simulink model "case5"  (R2024b)
settings: Solver=FixedStepAuto  StartTime=0  StopTime=1  FixedStep=1e-7  RelTol=1e-3
values from neighbouring files (symbols this model uses):
  SG_D_1_D = 0.01056    [IEEE9_case_parameters.m]    (also in case1_parameters.m; case2_parameters.m; case3_parameters.m; case4_parameters.m)
  SG_D_1_EnableSaturation = 0    [IEEE9_case_parameters.m]    (also in case1_parameters.m; case2_parameters.m; case3_parameters.m; case4_parameters.m)
  SG_D_1_f0 = 60    [IEEE9_case_parameters.m]    (also in case1_parameters.m; case2_parameters.m; case3_parameters.m; case4_parameters.m)
  SG_D_1_H = 7.5    [IEEE9_case_parameters.m]    (also in case1_parameters.m; case2_parameters.m; case3_parameters.m; case4_parameters.m)
  SG_D_1_K_A = 20    [IEEE9_case_parameters.m]    (also in case1_parameters.m; case2_parameters.m; case3_parameters.m; case4_parameters.m)
  SG_D_1_K_E = 1.000000e+1    (= 10)    [IEEE9_case_parameters.m]    (also in case1_parameters.m; case2_parameters.m; case3_parameters.m; case4_parameters.m)
  SG_D_1_K_F = 2.363    [IEEE9_case_parameters.m]    (also in case1_parameters.m; case2_parameters.m; case3_parameters.m; case4_parameters.m)
  SG_D_1_K_s = 0.5    [IEEE9_case_parameters.m]    (also in case1_parameters.m = 5; case2_parameters.m = 5; case3_parameters.m = 5; case4_parameters.m = 5)
  SG_D_1_R_a = 0.001088    [IEEE9_case_parameters.m]    (also in case1_parameters.m; case2_parameters.m; case3_parameters.m; case4_parameters.m)
  SG_D_1_S_A = 1    [IEEE9_case_parameters.m]    (also in case1_parameters.m; case2_parameters.m; case3_parameters.m; case4_parameters.m)
  SG_D_1_S_B = 0.103    [IEEE9_case_parameters.m]    (also in case1_parameters.m; case2_parameters.m; case3_parameters.m; case4_parameters.m)
  SG_D_1_S_N = 10.659857    [IEEE9_case_parameters.m]    (also in case1_parameters.m; case2_parameters.m; case3_parameters.m; case4_parameters.m)
  SG_D_1_SpeedPara = 200    [IEEE9_case_parameters.m]    (also in case1_parameters.m; case2_parameters.m; case3_parameters.m; case4_parameters.m)
  SG_D_1_T_0 = 0.720173    [IEEE9_case_parameters.m]    (also in case1_parameters.m = 0.755522; case2_parameters.m = 0.808931; case3_parameters.m = 0.869402; case4_parameters.m = 0.729316)
  SG_D_1_T_1 = 0.3    [IEEE9_case_parameters.m]    (also in case1_parameters.m; case2_parameters.m; case3_parameters.m; case4_parameters.m)
  SG_D_1_T_2 = 0.05    [IEEE9_case_parameters.m]    (also in case1_parameters.m; case2_parameters.m; case3_parameters.m; case4_parameters.m)
  SG_D_1_T_3 = 0.02    [IEEE9_case_parameters.m]    (also in case1_parameters.m; case2_parameters.m; case3_parameters.m; case4_parameters.m)
  SG_D_1_T_4 = 0.005    [IEEE9_case_parameters.m]    (also in case1_parameters.m; case2_parameters.m; case3_parameters.m; case4_parameters.m)
  SG_D_1_T_A = 0.02    [IEEE9_case_parameters.m]    (also in case1_parameters.m; case2_parameters.m; case3_parameters.m; case4_parameters.m)
  SG_D_1_T_dd = 8.000000e+0    (= 8)    [IEEE9_case_parameters.m]    (also in case1_parameters.m; case2_parameters.m; case3_parameters.m; case4_parameters.m)
  SG_D_1_T_ddd = 0.04    [IEEE9_case_parameters.m]    (also in case1_parameters.m; case2_parameters.m; case3_parameters.m; case4_parameters.m)
  SG_D_1_T_E = 0.314    [IEEE9_case_parameters.m]    (also in case1_parameters.m; case2_parameters.m; case3_parameters.m; case4_parameters.m)
  SG_D_1_T_F = 0.35    [IEEE9_case_parameters.m]    (also in case1_parameters.m; case2_parameters.m; case3_parameters.m; case4_parameters.m)
  SG_D_1_T_qd = 0.8    [IEEE9_case_parameters.m]    (also in case1_parameters.m; case2_parameters.m; case3_parameters.m; case4_parameters.m)
  SG_D_1_T_qdd = 0.02    [IEEE9_case_parameters.m]    (also in case1_parameters.m; case2_parameters.m; case3_parameters.m; case4_parameters.m)
  SG_D_1_T_speed = 0.1    [IEEE9_case_parameters.m]    (also in case1_parameters.m = 200; case2_parameters.m = 200; case3_parameters.m = 200; case4_parameters.m = 200)
  SG_D_1_T_w = 0.5    [IEEE9_case_parameters.m]    (also in case1_parameters.m; case2_parameters.m; case3_parameters.m; case4_parameters.m)
  SG_D_1_V_ref = 1.990276    [IEEE9_case_parameters.m]    (also in case1_parameters.m = 2.042296; case2_parameters.m = 2.051388; case3_parameters.m = 2.089584; case4_parameters.m = 2.01845)
  SG_D_1_w_ref = 376.991118    [IEEE9_case_parameters.m]    (also in case1_parameters.m; case2_parameters.m; case3_parameters.m; case4_parameters.m)
  SG_D_1_wb = 6.000000e+1    (= 60)    [IEEE9_case_parameters.m]    (also in case1_parameters.m; case2_parameters.m; case3_parameters.m; case4_parameters.m)
  SG_D_1_x_d = 1.9    [IEEE9_case_parameters.m]    (also in case1_parameters.m; case2_parameters.m; case3_parameters.m; case4_parameters.m)
  SG_D_1_x_dd = 0.302    [IEEE9_case_parameters.m]    (also in case1_parameters.m; case2_parameters.m; case3_parameters.m; case4_parameters.m)
  SG_D_1_x_ddd = 0.204    [IEEE9_case_parameters.m]    (also in case1_parameters.m; case2_parameters.m; case3_parameters.m; case4_parameters.m)
  SG_D_1_x_l = 0.05    [IEEE9_case_parameters.m]    (also in case1_parameters.m; case2_parameters.m; case3_parameters.m; case4_parameters.m)
  SG_D_1_x_q = 1.3    [IEEE9_case_parameters.m]    (also in case1_parameters.m; case2_parameters.m; case3_parameters.m; case4_parameters.m)
  SG_D_1_x_qd = 0.5    [IEEE9_case_parameters.m]    (also in case1_parameters.m; case2_parameters.m; case3_parameters.m; case4_parameters.m)
  SG_D_1_x_qdd = 0.3    [IEEE9_case_parameters.m]    (also in case1_parameters.m; case2_parameters.m; case3_parameters.m; case4_parameters.m)
  SG_D_2_D = 0.02    [IEEE9_case_parameters.m]    (also in case1_parameters.m; case2_parameters.m; case3_parameters.m; case4_parameters.m)
  SG_D_2_EnableSaturation = 0    [IEEE9_case_parameters.m]    (also in case1_parameters.m; case2_parameters.m; case3_parameters.m; case4_parameters.m)
  SG_D_2_f0 = 60    [IEEE9_case_parameters.m]    (also in case1_parameters.m; case2_parameters.m; case3_parameters.m; case4_parameters.m)
  SG_D_2_H = 8.000000e+0    (= 8)    [IEEE9_case_parameters.m]    (also in case1_parameters.m; case2_parameters.m; case3_parameters.m; case4_parameters.m)
  SG_D_2_K_A = 20    [IEEE9_case_parameters.m]    (also in case1_parameters.m; case2_parameters.m; case3_parameters.m; case4_parameters.m)
  SG_D_2_K_E = 1.000000e+1    (= 10)    [IEEE9_case_parameters.m]    (also in case1_parameters.m; case2_parameters.m; case3_parameters.m; case4_parameters.m)
  SG_D_2_K_F = 2.363    [IEEE9_case_parameters.m]    (also in case1_parameters.m; case2_parameters.m; case3_parameters.m; case4_parameters.m)
  SG_D_2_K_s = 0.5    [IEEE9_case_parameters.m]    (also in case1_parameters.m = 4; case2_parameters.m = 4; case3_parameters.m = 4; case4_parameters.m = 4)
  SG_D_2_R_a = 0.001088    [IEEE9_case_parameters.m]    (also in case1_parameters.m; case2_parameters.m; case3_parameters.m; case4_parameters.m)
  SG_D_2_S_A = 1    [IEEE9_case_parameters.m]    (also in case1_parameters.m; case2_parameters.m; case3_parameters.m; case4_parameters.m)
  SG_D_2_S_B = 0.103    [IEEE9_case_parameters.m]    (also in case1_parameters.m; case2_parameters.m; case3_parameters.m; case4_parameters.m)
  SG_D_2_S_N = 10.659857    [IEEE9_case_parameters.m]    (also in case1_parameters.m; case2_parameters.m; case3_parameters.m; case4_parameters.m)
  SG_D_2_SpeedPara = 200    [IEEE9_case_parameters.m]    (also in case1_parameters.m; case2_parameters.m; case3_parameters.m; case4_parameters.m)
  SG_D_2_T_0 = 1.632913    [IEEE9_case_parameters.m]    (also in case1_parameters.m = 1.632925; case2_parameters.m = 1.632915; case3_parameters.m = 1.632914; case4_parameters.m = 1.632927)
  SG_D_2_T_1 = 0.2    [IEEE9_case_parameters.m]    (also in case1_parameters.m; case2_parameters.m; case3_parameters.m; case4_parameters.m)
  SG_D_2_T_2 = 0.05    [IEEE9_case_parameters.m]    (also in case1_parameters.m; case2_parameters.m; case3_parameters.m; case4_parameters.m)
  SG_D_2_T_3 = 0.02    [IEEE9_case_parameters.m]    (also in case1_parameters.m; case2_parameters.m; case3_parameters.m; case4_parameters.m)
  SG_D_2_T_4 = 0.005    [IEEE9_case_parameters.m]    (also in case1_parameters.m; case2_parameters.m; case3_parameters.m; case4_parameters.m)
  SG_D_2_T_A = 0.02    [IEEE9_case_parameters.m]    (also in case1_parameters.m; case2_parameters.m; case3_parameters.m; case4_parameters.m)
  SG_D_2_T_dd = 7.9    [IEEE9_case_parameters.m]    (also in case1_parameters.m; case2_parameters.m; case3_parameters.m; case4_parameters.m)
  SG_D_2_T_ddd = 0.04    [IEEE9_case_parameters.m]    (also in case1_parameters.m; case2_parameters.m; case3_parameters.m; case4_parameters.m)
  SG_D_2_T_E = 0.314    [IEEE9_case_parameters.m]    (also in case1_parameters.m; case2_parameters.m; case3_parameters.m; case4_parameters.m)
  SG_D_2_T_F = 0.35    [IEEE9_case_parameters.m]    (also in case1_parameters.m; case2_parameters.m; case3_parameters.m; case4_parameters.m)
  SG_D_2_T_qd = 0.8    [IEEE9_case_parameters.m]    (also in case1_parameters.m; case2_parameters.m; case3_parameters.m; case4_parameters.m)
  SG_D_2_T_qdd = 0.015    [IEEE9_case_parameters.m]    (also in case1_parameters.m; case2_parameters.m; case3_parameters.m; case4_parameters.m)
  SG_D_2_T_speed = 0.1    [IEEE9_case_parameters.m]    (also in case1_parameters.m = 150; case2_parameters.m = 150; case3_parameters.m = 150; case4_parameters.m = 150)
  SG_D_2_T_w = 0.35    [IEEE9_case_parameters.m]    (also in case1_parameters.m; case2_parameters.m; case3_parameters.m; case4_parameters.m)
  SG_D_2_V_ref = 2.58547    [IEEE9_case_parameters.m]    (also in case1_parameters.m = 2.597896; case2_parameters.m = 2.587136; case3_parameters.m = 2.586042; case4_parameters.m = 2.599679)
  SG_D_2_w_ref = 376.991118    [IEEE9_case_parameters.m]    (also in case1_parameters.m; case2_parameters.m; case3_parameters.m; case4_parameters.m)
  SG_D_2_wb = 6.000000e+1    (= 60)    [IEEE9_case_parameters.m]    (also in case1_parameters.m; case2_parameters.m; case3_parameters.m; case4_parameters.m)
  SG_D_2_x_d = 1.8    [IEEE9_case_parameters.m]    (also in case1_parameters.m; case2_parameters.m; case3_parameters.m; case4_parameters.m)
  SG_D_2_x_dd = 0.302    [IEEE9_case_parameters.m]    (also in case1_parameters.m; case2_parameters.m; case3_parameters.m; case4_parameters.m)
  SG_D_2_x_ddd = 0.204    [IEEE9_case_parameters.m]    (also in case1_parameters.m; case2_parameters.m; case3_parameters.m; case4_parameters.m)
  SG_D_2_x_l = 0.05    [IEEE9_case_parameters.m]    (also in case1_parameters.m; case2_parameters.m; case3_parameters.m; case4_parameters.m)
  SG_D_2_x_q = 1.25    [IEEE9_case_parameters.m]    (also in case1_parameters.m; case2_parameters.m; case3_parameters.m; case4_parameters.m)
  SG_D_2_x_qd = 0.5    [IEEE9_case_parameters.m]    (also in case1_parameters.m; case2_parameters.m; case3_parameters.m; case4_parameters.m)
  SG_D_2_x_qdd = 0.3    [IEEE9_case_parameters.m]    (also in case1_parameters.m; case2_parameters.m; case3_parameters.m; case4_parameters.m)
  SG_D_3_D = 0.02    [IEEE9_case_parameters.m]    (also in case1_parameters.m; case2_parameters.m; case3_parameters.m; case4_parameters.m)
  SG_D_3_EnableSaturation = 0    [IEEE9_case_parameters.m]    (also in case1_parameters.m; case2_parameters.m; case3_parameters.m; case4_parameters.m)
  SG_D_3_f0 = 60    [IEEE9_case_parameters.m]    (also in case1_parameters.m; case2_parameters.m; case3_parameters.m; case4_parameters.m)
  SG_D_3_H = 7.7    [IEEE9_case_parameters.m]    (also in case1_parameters.m; case2_parameters.m; case3_parameters.m; case4_parameters.m)
  SG_D_3_K_A = 20    [IEEE9_case_parameters.m]    (also in case1_parameters.m; case2_parameters.m; case3_parameters.m; case4_parameters.m)
  SG_D_3_K_E = 1.000000e+1    (= 10)    [IEEE9_case_parameters.m]    (also in case1_parameters.m; case2_parameters.m; case3_parameters.m; case4_parameters.m)
  SG_D_3_K_F = 2.363    [IEEE9_case_parameters.m]    (also in case1_parameters.m; case2_parameters.m; case3_parameters.m; case4_parameters.m)
  SG_D_3_K_s = 0.2    [IEEE9_case_parameters.m]    (also in case1_parameters.m = 2; case2_parameters.m = 2; case3_parameters.m = 2; case4_parameters.m = 2)
  SG_D_3_R_a = 0.001088    [IEEE9_case_parameters.m]    (also in case1_parameters.m; case2_parameters.m; case3_parameters.m; case4_parameters.m)
  SG_D_3_S_A = 1    [IEEE9_case_parameters.m]    (also in case1_parameters.m; case2_parameters.m; case3_parameters.m; case4_parameters.m)
  SG_D_3_S_B = 0.103    [IEEE9_case_parameters.m]    (also in case1_parameters.m; case2_parameters.m; case3_parameters.m; case4_parameters.m)
  SG_D_3_S_N = 10.659857    [IEEE9_case_parameters.m]    (also in case1_parameters.m; case2_parameters.m; case3_parameters.m; case4_parameters.m)
  SG_D_3_SpeedPara = 200    [IEEE9_case_parameters.m]    (also in case1_parameters.m; case2_parameters.m; case3_parameters.m; case4_parameters.m)
  SG_D_3_T_0 = 0.850788    [IEEE9_case_parameters.m]    (also in case1_parameters.m = 0.850786; case2_parameters.m = 0.850787; case3_parameters.m; case4_parameters.m = 0.850786)
  SG_D_3_T_1 = 0.2    [IEEE9_case_parameters.m]    (also in case1_parameters.m; case2_parameters.m; case3_parameters.m; case4_parameters.m)
  SG_D_3_T_2 = 0.05    [IEEE9_case_parameters.m]    (also in case1_parameters.m; case2_parameters.m; case3_parameters.m; case4_parameters.m)
  SG_D_3_T_3 = 0.02    [IEEE9_case_parameters.m]    (also in case1_parameters.m; case2_parameters.m; case3_parameters.m; case4_parameters.m)
  SG_D_3_T_4 = 0.005    [IEEE9_case_parameters.m]    (also in case1_parameters.m; case2_parameters.m; case3_parameters.m; case4_parameters.m)
  SG_D_3_T_A = 0.02    [IEEE9_case_parameters.m]    (also in case1_parameters.m; case2_parameters.m; case3_parameters.m; case4_parameters.m)
  SG_D_3_T_dd = 8.1    [IEEE9_case_parameters.m]    (also in case1_parameters.m; case2_parameters.m; case3_parameters.m; case4_parameters.m)
  SG_D_3_T_ddd = 0.04    [IEEE9_case_parameters.m]    (also in case1_parameters.m; case2_parameters.m; case3_parameters.m; case4_parameters.m)
  SG_D_3_T_E = 0.314    [IEEE9_case_parameters.m]    (also in case1_parameters.m; case2_parameters.m; case3_parameters.m; case4_parameters.m)
  SG_D_3_T_F = 0.35    [IEEE9_case_parameters.m]    (also in case1_parameters.m; case2_parameters.m; case3_parameters.m; case4_parameters.m)
  SG_D_3_T_qd = 0.8    [IEEE9_case_parameters.m]    (also in case1_parameters.m; case2_parameters.m; case3_parameters.m; case4_parameters.m)
  SG_D_3_T_qdd = 0.015    [IEEE9_case_parameters.m]    (also in case1_parameters.m; case2_parameters.m; case3_parameters.m; case4_parameters.m)
  SG_D_3_T_speed = 0.1    [IEEE9_case_parameters.m]    (also in case1_parameters.m = 180; case2_parameters.m = 180; case3_parameters.m = 180; case4_parameters.m = 180)
  SG_D_3_T_w = 0.4    [IEEE9_case_parameters.m]    (also in case1_parameters.m; case2_parameters.m; case3_parameters.m; case4_parameters.m)
  SG_D_3_V_ref = 1.892727    [IEEE9_case_parameters.m]    (also in case1_parameters.m = 1.906439; case2_parameters.m = 1.895535; case3_parameters.m = 1.892105; case4_parameters.m = 1.906598)
  SG_D_3_w_ref = 376.991118    [IEEE9_case_parameters.m]    (also in case1_parameters.m; case2_parameters.m; case3_parameters.m; case4_parameters.m)
  SG_D_3_wb = 6.000000e+1    (= 60)    [IEEE9_case_parameters.m]    (also in case1_parameters.m; case2_parameters.m; case3_parameters.m; case4_parameters.m)
  SG_D_3_x_d = 1.85    [IEEE9_case_parameters.m]    (also in case1_parameters.m; case2_parameters.m; case3_parameters.m; case4_parameters.m)
  SG_D_3_x_dd = 0.302    [IEEE9_case_parameters.m]    (also in case1_parameters.m; case2_parameters.m; case3_parameters.m; case4_parameters.m)
  SG_D_3_x_ddd = 0.204    [IEEE9_case_parameters.m]    (also in case1_parameters.m; case2_parameters.m; case3_parameters.m; case4_parameters.m)
  SG_D_3_x_l = 0.05    [IEEE9_case_parameters.m]    (also in case1_parameters.m; case2_parameters.m; case3_parameters.m; case4_parameters.m)
  SG_D_3_x_q = 1.2    [IEEE9_case_parameters.m]    (also in case1_parameters.m; case2_parameters.m; case3_parameters.m; case4_parameters.m)
  SG_D_3_x_qd = 0.5    [IEEE9_case_parameters.m]    (also in case1_parameters.m; case2_parameters.m; case3_parameters.m; case4_parameters.m)
  SG_D_3_x_qdd = 0.3    [IEEE9_case_parameters.m]    (also in case1_parameters.m; case2_parameters.m; case3_parameters.m; case4_parameters.m)
(part 8 of 12)

== system case5/SG_D_2/d_psi_d_SG_D_2_block ==
  note: d_psi_d_SG_D_2 in case5
      | $2\,\pi \,f_{0}\,\left(v_{d,\mathrm{SG},D,2}\,\sin\left(\theta _{\mathrm{SG},D,2}\right)-v_{q,\mathrm{SG},D,2}\,\cos\left(\theta _{\mathrm{SG},D,2}\right)+\frac{R_{a}\,\left(\frac{\psi _{\mathrm{1d},\mathrm{SG},D,2}\,\left(x_{\mathrm{dd}}-x_{\mathrm{ddd}}\right)}{x_{\mathrm{dd}}-x_{l}}-\psi _{d,\mathrm{SG},D,2}+\frac{\psi _{\mathrm{fd},\mathrm{SG},D,2}\,\left(x_{\mathrm{ddd}}-x_{l}\right)}{x_{\mathrm{dd}}-x_{l}}\right)}{x_{\mathrm{ddd}}}+\frac{\psi _{q,\mathrm{SG},D,2}\,w_{\mathrm{SG},D,2}}{2\,f_{0}\,\pi }\right)$
      | Automatically generated on 2025-10-31 19:10:55 .
  State_psi_1d_SG_D_2_04eff : Inport
  State_psi_d_SG_D_2_38234 : Inport  Port=2
  State_psi_fd_SG_D_2_ff9ed : Inport  Port=3
  Input_v_d_SG_D_2_e8182 : Inport  Port=4
  State_theta_SG_D_2_47dce : Inport  Port=5
  Input_v_q_SG_D_2_617bb : Inport  Port=6
  State_theta_SG_D_2_18c28 : Inport  Port=7
  State_psi_q_SG_D_2_39081 : Inport  Port=8
  State_w_SG_D_2_93911 : Inport  Port=9
  Add_35a87 : Sum
  Add_8a6e8 : Sum
  Constant_-1_40228 : Constant  Value=-1
  Constant_-2.0_2b37e : Constant  Value=-2.0
  Constant_2.0_61fa9 : Constant  Value=2.0
  Constant_R_a_dc03f : Constant  Value=R_a
  Constant_f0_9e30f : Constant  Value=f0
  Constant_f0_ea738 : Constant  Value=f0
  Constant_pi_80db8 : Constant  Value=pi
  Constant_pi_cc7e5 : Constant  Value=pi
  Constant_x_dd_383e0 : Constant  Value=x_dd
  Constant_x_dd_5a803 : Constant  Value=x_dd
  Constant_x_dd_d00b2 : Constant  Value=x_dd
  Constant_x_ddd_020f5 : Constant  Value=x_ddd
  Constant_x_ddd_24d94 : Constant  Value=x_ddd
  Constant_x_ddd_dd370 : Constant  Value=x_ddd
  Constant_x_l_7a989 : Constant  Value=x_l
  Constant_x_l_d2dea : Constant  Value=x_l
  Constant_x_l_e9755 : Constant  Value=x_l
  Divide_2b41b : Product  Inputs=*/
  Divide_53e77 : Product  Inputs=*/
  Divide_973af : Product  Inputs=*/
  Divide_a5896 : Product  Inputs=*/
  MathFunc_cos_96fd6 : Trigonometry  Operator=cos
  MathFunc_sin_6bfeb : Trigonometry
  Product_21970 : Product
  Product_5265e : Product
  Product_60fe7 : Product
  Product_61b83 : Product
  Product_79863 : Product
  Product_8e8bd : Product
  Product_ab31f : Product
  Product_caa64 : Product
  Product_cea4f : Product
  Product_d6891 : Product
  Product_e49bf : Product
  Product_fc14d : Product
  Subtract_54247 : Sum  Inputs=+-
  Subtract_54db2 : Sum  Inputs=+-
  Subtract_7347e : Sum  Inputs=+-
  Subtract_9dfb5 : Sum  Inputs=+-
  Subtract_e25de : Sum  Inputs=+-
  Subtract_e48e5 : Sum  Inputs=+-
  Subtract_f9a11 : Sum  Inputs=+-
  Blockout_d_psi_d_SG_D_2_c5ec0 : Outport
  wires:
  MathFunc_sin_6bfeb/1 -> Product_d6891/2
  Constant_x_dd_d00b2/1 -> Subtract_9dfb5/1
  Constant_-1_40228/1 -> Product_8e8bd/1
  Constant_x_l_d2dea/1 -> Subtract_9dfb5/2
  State_psi_1d_SG_D_2_04eff/1 -> Product_8e8bd/2
  Constant_f0_ea738/1 -> Product_5265e/2
  Constant_2.0_61fa9/1 -> Product_e49bf/1
  Constant_x_l_e9755/1 -> Subtract_f9a11/2
  Constant_x_dd_5a803/1 -> Subtract_54db2/1
  Product_60fe7/1 -> Blockout_d_psi_d_SG_D_2_c5ec0/1
  Constant_pi_cc7e5/1 -> Product_e49bf/2
  Constant_x_ddd_020f5/1 -> Subtract_54db2/2
  Subtract_e48e5/1 -> Product_60fe7/2
  Product_8e8bd/1 -> Product_caa64/1
  Product_e49bf/1 -> Product_61b83/1
  Subtract_54db2/1 -> Product_caa64/2
  Divide_a5896/1 -> Subtract_e48e5/2
  Constant_x_ddd_24d94/1 -> Subtract_e25de/1
  Constant_x_l_7a989/1 -> Subtract_e25de/2
  Product_caa64/1 -> Divide_53e77/1
  Subtract_54247/1 -> Add_8a6e8/1
  Subtract_9dfb5/1 -> Divide_53e77/2
  State_psi_fd_SG_D_2_ff9ed/1 -> Product_fc14d/1
  Subtract_e25de/1 -> Product_fc14d/2
  Constant_x_dd_383e0/1 -> Subtract_f9a11/1
  Divide_53e77/1 -> Add_35a87/1
  State_psi_d_SG_D_2_38234/1 -> Add_35a87/2
  Product_fc14d/1 -> Divide_2b41b/1
  Subtract_f9a11/1 -> Divide_2b41b/2
  Add_35a87/1 -> Subtract_7347e/1
  Divide_2b41b/1 -> Subtract_7347e/2
  Constant_R_a_dc03f/1 -> Product_ab31f/1
  Subtract_7347e/1 -> Product_ab31f/2
  Divide_973af/1 -> Subtract_54247/1
  State_theta_SG_D_2_47dce/1 -> MathFunc_sin_6bfeb/1
  Product_ab31f/1 -> Divide_973af/1
  Constant_-2.0_2b37e/1 -> Product_79863/1
  Input_v_d_SG_D_2_e8182/1 -> Product_d6891/1
  Constant_x_ddd_dd370/1 -> Divide_973af/2
  State_theta_SG_D_2_18c28/1 -> MathFunc_cos_96fd6/1
  Product_5265e/1 -> Product_60fe7/1
  Product_d6891/1 -> Subtract_54247/2
  Product_79863/1 -> Product_5265e/1
  Input_v_q_SG_D_2_617bb/1 -> Product_cea4f/1
  MathFunc_cos_96fd6/1 -> Product_cea4f/2
  State_psi_q_SG_D_2_39081/1 -> Product_21970/1
  State_w_SG_D_2_93911/1 -> Product_21970/2
  Constant_f0_9e30f/1 -> Product_61b83/2
  Constant_pi_80db8/1 -> Product_79863/2
  Product_cea4f/1 -> Add_8a6e8/2
  Product_21970/1 -> Divide_a5896/1
  Product_61b83/1 -> Divide_a5896/2
  Add_8a6e8/1 -> Subtract_e48e5/1

== system case5/SG_D_2/d_psi_fd_SG_D_2_block ==
  note: d_psi_fd_SG_D_2 in case5
      | $-\frac{\psi _{\mathrm{fd},\mathrm{SG},D,2}-E_{\mathrm{fd},\mathrm{SG},D,2}+\left(x_{d}-x_{\mathrm{dd}}\right)\,\left(\frac{\frac{\psi _{\mathrm{1d},\mathrm{SG},D,2}\,\left(x_{\mathrm{dd}}-x_{\mathrm{ddd}}\right)}{x_{\mathrm{dd}}-x_{l}}-\psi _{d,\mathrm{SG},D,2}+\frac{\psi _{\mathrm{fd},\mathrm{SG},D,2}\,\left(x_{\mathrm{ddd}}-x_{l}\right)}{x_{\mathrm{dd}}-x_{l}}}{x_{\mathrm{ddd}}}-\frac{\left(x_{\mathrm{dd}}-x_{\mathrm{ddd}}\right)\,\left(\psi _{\mathrm{1d},\mathrm{SG},D,2}-\psi _{\mathrm{fd},\mathrm{SG},D,2}+\frac{\left(x_{\mathrm{dd}}-x_{l}\right)\,\left(\frac{\psi _{\mathrm{1d},\mathrm{SG},D,2}\,\left(x_{\mathrm{dd}}-x_{\mathrm{ddd}}\right)}{x_{\mathrm{dd}}-x_{l}}-\psi _{d,\mathrm{SG},D,2}+\frac{\psi _{\mathrm{fd},\mathrm{SG},D,2}\,\left(x_{\mathrm{ddd}}-x_{l}\right)}{x_{\mathrm{dd}}-x_{l}}\right)}{x_{\mathrm{ddd}}}\right)}{{\left(x_{\mathrm{dd}}-x_{l}\right)}^2}\right)}{T_{\mathrm{dd}}}$
      | Automatically generated on 2025-10-31 19:11:05 .
  State_E_fd_SG_D_2_4bfea : Inport
  State_psi_fd_SG_D_2_52249 : Inport  Port=2
  State_psi_1d_SG_D_2_569a8 : Inport  Port=3
  State_psi_fd_SG_D_2_bd521 : Inport  Port=4
  State_psi_1d_SG_D_2_de869 : Inport  Port=5
  State_psi_d_SG_D_2_2ae43 : Inport  Port=6
  State_psi_fd_SG_D_2_2448d : Inport  Port=7
  State_psi_1d_SG_D_2_50b72 : Inport  Port=8
  State_psi_d_SG_D_2_60bb1 : Inport  Port=9
  State_psi_fd_SG_D_2_29cbb : Inport  Port=10
  Add_807b0 : Sum
  Add_92990 : Sum
  Constant_-1_18d3b : Constant  Value=-1
  Constant_-1_23845 : Constant  Value=-1
  Constant_-1_3a1c2 : Constant  Value=-1
  Constant_2.0_fae6e : Constant  Value=2.0
  Constant_T_dd_c2c29 : Constant  Value=T_dd
  Constant_x_d_43747 : Constant  Value=x_d
  Constant_x_dd_10bf3 : Constant  Value=x_dd
  Constant_x_dd_24d9e : Constant  Value=x_dd
  Constant_x_dd_261bc : Constant  Value=x_dd
  Constant_x_dd_4acb3 : Constant  Value=x_dd
  Constant_x_dd_c1aff : Constant  Value=x_dd
  Constant_x_dd_cff65 : Constant  Value=x_dd
  Constant_x_dd_d5cdf : Constant  Value=x_dd
  Constant_x_dd_dae7c : Constant  Value=x_dd
  Constant_x_dd_f7268 : Constant  Value=x_dd
  Constant_x_dd_fe35d : Constant  Value=x_dd
  Constant_x_ddd_0888f : Constant  Value=x_ddd
  Constant_x_ddd_124ec : Constant  Value=x_ddd
  Constant_x_ddd_44805 : Constant  Value=x_ddd
  Constant_x_ddd_7c7c3 : Constant  Value=x_ddd
  Constant_x_ddd_a1edb : Constant  Value=x_ddd
  Constant_x_ddd_a6cd1 : Constant  Value=x_ddd
  Constant_x_ddd_c2edf : Constant  Value=x_ddd
  Constant_x_l_59093 : Constant  Value=x_l
  Constant_x_l_768d7 : Constant  Value=x_l
  Constant_x_l_7bddd : Constant  Value=x_l
  Constant_x_l_92fb9 : Constant  Value=x_l
  Constant_x_l_b5f95 : Constant  Value=x_l
  Constant_x_l_ca421 : Constant  Value=x_l
  Constant_x_l_cff4a : Constant  Value=x_l
  Constant_x_l_d3abc : Constant  Value=x_l
  Divide_46224 : Product  Inputs=*/
  Divide_4a4ac : Product  Inputs=*/
  Divide_67d0a : Product  Inputs=*/
  Divide_6e8e2 : Product  Inputs=*/
  Divide_7626a : Product  Inputs=*/
  Divide_8d5c8 : Product  Inputs=*/
  Divide_c3267 : Product  Inputs=*/
  Divide_c3f1b : Product  Inputs=*/
  Power_391a0 : Math  Operator=pow
  Product_271b3 : Product
  Product_461f0 : Product
  Product_624bd : Product
  Product_95ff3 : Product
  Product_b9362 : Product
  Product_baa0b : Product
  Product_d2126 : Product
  Product_eaf31 : Product
  Product_f9a51 : Product
  Product_ff220 : Product
  Subtract_01693 : Sum  Inputs=+-
  Subtract_099c9 : Sum  Inputs=+-
  Subtract_0f381 : Sum  Inputs=+-
  Subtract_17e32 : Sum  Inputs=+-
  Subtract_25243 : Sum  Inputs=+-
  Subtract_283d9 : Sum  Inputs=+-
  Subtract_2ee32 : Sum  Inputs=+-
  Subtract_301a9 : Sum  Inputs=+-
  Subtract_3e025 : Sum  Inputs=+-
  Subtract_74e66 : Sum  Inputs=+-
  Subtract_79f9a : Sum  Inputs=+-
  Subtract_8fe35 : Sum  Inputs=+-
  Subtract_9ac67 : Sum  Inputs=+-
  Subtract_ab91b : Sum  Inputs=+-
  Subtract_b343b : Sum  Inputs=+-
  Subtract_bbb0c : Sum  Inputs=+-
  Subtract_d8d56 : Sum  Inputs=+-
  Subtract_dd31b : Sum  Inputs=+-
  Subtract_e919c : Sum  Inputs=+-
  Blockout_d_psi_fd_SG_D_2_6ca49 : Outport
  wires:
  Constant_x_dd_cff65/1 -> Subtract_b343b/1
  Constant_-1_3a1c2/1 -> Product_eaf31/1
  Constant_x_l_d3abc/1 -> Subtract_ab91b/2
  Divide_46224/1 -> Add_807b0/1
  Subtract_099c9/1 -> Product_ff220/2
  Constant_x_l_768d7/1 -> Subtract_b343b/2
  Product_ff220/1 -> Divide_4a4ac/1
  State_psi_1d_SG_D_2_de869/1 -> Product_eaf31/2
  Constant_x_dd_f7268/1 -> Subtract_2ee32/1
  Product_461f0/1 -> Divide_46224/1
  Constant_x_dd_d5cdf/1 -> Subtract_0f381/1
  Constant_x_ddd_124ec/1 -> Subtract_2ee32/2
  Constant_x_dd_261bc/1 -> Subtract_dd31b/1
  Product_eaf31/1 -> Product_b9362/1
  Subtract_2ee32/1 -> Product_b9362/2
  State_psi_d_SG_D_2_60bb1/1 -> Add_807b0/2
  Constant_x_ddd_a1edb/1 -> Subtract_099c9/1
  Constant_x_l_59093/1 -> Subtract_099c9/2
  Product_b9362/1 -> Divide_c3267/1
  Subtract_b343b/1 -> Divide_c3267/2
  State_psi_fd_SG_D_2_2448d/1 -> Product_ff220/1
  Subtract_79f9a/1 -> Product_d2126/2
  Constant_x_dd_24d9e/1 -> Subtract_e919c/1
  Constant_x_l_7bddd/1 -> Subtract_e919c/2
  Product_624bd/1 -> Product_d2126/1
  Divide_c3267/1 -> Add_92990/1
  State_psi_d_SG_D_2_2ae43/1 -> Add_92990/2
  Subtract_e919c/1 -> Divide_4a4ac/2
  Constant_x_dd_fe35d/1 -> Subtract_ab91b/1
  Constant_x_ddd_a6cd1/1 -> Subtract_01693/1
  Add_92990/1 -> Subtract_17e32/1
  Divide_4a4ac/1 -> Subtract_17e32/2
  Constant_-1_23845/1 -> Product_baa0b/1
  Product_95ff3/1 -> Divide_7626a/1
  State_psi_1d_SG_D_2_50b72/1 -> Product_baa0b/2
  Subtract_0f381/1 -> Product_624bd/2
  Constant_x_dd_4acb3/1 -> Subtract_d8d56/1
  Divide_7626a/1 -> Subtract_8fe35/2
  Constant_-1_18d3b/1 -> Product_624bd/1
  Constant_x_ddd_c2edf/1 -> Subtract_d8d56/2
  Constant_x_ddd_0888f/1 -> Divide_6e8e2/2
  Subtract_ab91b/1 -> Product_271b3/1
  Subtract_17e32/1 -> Product_271b3/2
  State_psi_fd_SG_D_2_bd521/1 -> Subtract_9ac67/2
  Product_baa0b/1 -> Product_461f0/1
  Subtract_d8d56/1 -> Product_461f0/2
  Constant_2.0_fae6e/1 -> Power_391a0/2
  State_psi_1d_SG_D_2_569a8/1 -> Subtract_9ac67/1
  Constant_x_dd_dae7c/1 -> Subtract_301a9/1
  Subtract_01693/1 -> Product_95ff3/2
  Constant_x_l_ca421/1 -> Subtract_301a9/2
  Constant_x_l_cff4a/1 -> Subtract_01693/2
  Constant_x_ddd_44805/1 -> Subtract_0f381/2
  Subtract_dd31b/1 -> Divide_7626a/2
  Product_271b3/1 -> Divide_6e8e2/1
  Subtract_301a9/1 -> Divide_46224/2
  State_psi_fd_SG_D_2_29cbb/1 -> Product_95ff3/1
  Constant_x_l_b5f95/1 -> Subtract_dd31b/2
  Constant_x_dd_10bf3/1 -> Subtract_bbb0c/1
  Subtract_9ac67/1 -> Subtract_79f9a/1
  Divide_6e8e2/1 -> Subtract_79f9a/2
  Constant_x_l_92fb9/1 -> Subtract_bbb0c/2
  Subtract_bbb0c/1 -> Power_391a0/1
  Add_807b0/1 -> Subtract_8fe35/1
  Product_d2126/1 -> Divide_c3f1b/1
  Power_391a0/1 -> Divide_c3f1b/2
  Subtract_8fe35/1 -> Divide_8d5c8/1
  Constant_x_ddd_7c7c3/1 -> Divide_8d5c8/2
  Constant_x_d_43747/1 -> Subtract_25243/1
  Constant_x_dd_c1aff/1 -> Subtract_25243/2
  Divide_c3f1b/1 -> Subtract_283d9/1
  Divide_8d5c8/1 -> Subtract_283d9/2
  State_E_fd_SG_D_2_4bfea/1 -> Subtract_3e025/1
  State_psi_fd_SG_D_2_52249/1 -> Subtract_3e025/2
  Subtract_25243/1 -> Product_f9a51/1
  Subtract_283d9/1 -> Product_f9a51/2
  Subtract_3e025/1 -> Subtract_74e66/1
  Product_f9a51/1 -> Subtract_74e66/2
  Subtract_74e66/1 -> Divide_67d0a/1
  Constant_T_dd_c2c29/1 -> Divide_67d0a/2
  Divide_67d0a/1 -> Blockout_d_psi_fd_SG_D_2_6ca49/1

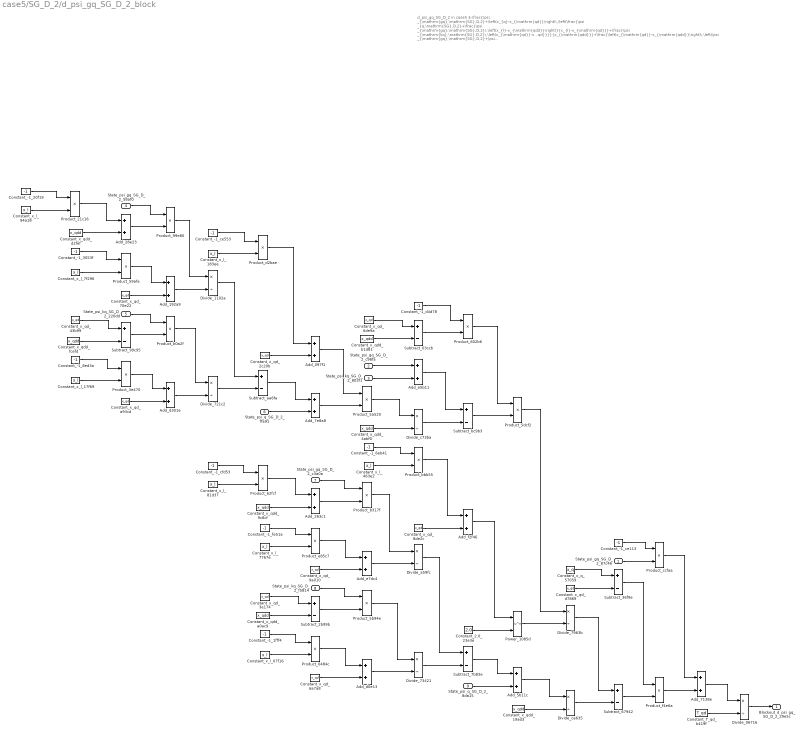
== system case5/SG_D_2/d_psi_gq_SG_D_2_block ==
  note: d_psi_gq_SG_D_2 in case5
      | $-\frac{\psi _{\mathrm{gq},\mathrm{SG},D,2}+\left(x_{q}-x_{\mathrm{qd}}\right)\,\left(\frac{\psi _{q,\mathrm{SG},D,2}+\frac{\psi _{\mathrm{gq},\mathrm{SG},D,2}\,\left(x_{l}-x_{\mathrm{qdd}}\right)}{x_{l}-x_{\mathrm{qd}}}+\frac{\psi _{\mathrm{kq},\mathrm{SG},D,2}\,\left(x_{\mathrm{qd}}-x_{\mathrm{qdd}}\right)}{x_{l}-x_{\mathrm{qd}}}}{x_{\mathrm{qdd}}}+\frac{\left(x_{\mathrm{qd}}-x_{\mathrm{qdd}}\right)\,\left(\psi _{\mathrm{gq},\mathrm{SG},D,2}+\psi _{\mathrm{kq},\mathrm{SG},D,2}+\frac{\left(x_{l}-x_{\mathrm{qd}}\right)\,\left(\psi _{q,\mathrm{SG},D,2}+\frac{\psi _{\mathrm{gq},\mathrm{SG},D,2}\,\left(x_{l}-x_{\mathrm{qdd}}\right)}{x_{l}-x_{\mathrm{qd}}}+\frac{\psi _{\mathrm{kq},\mathrm{SG},D,2}\,\left(x_{\mathrm{qd}}-x_{\mathrm{qdd}}\right)}{x_{l}-x_{\mathrm{qd}}}\right)}{x_{\mathrm{qdd}}}\right)}{{\left(x_{l}-x_{\mathrm{qd}}\right)}^2}\right)}{T_{\mathrm{qd}}}$
      | Automatically generated on 2025-10-31 19:11:15 .
  State_psi_gq_SG_D_2_87c46 : Inport
  State_psi_gq_SG_D_2_c98fa : Inport  Port=2
  State_psi_kq_SG_D_2_803f1 : Inport  Port=3
  State_psi_gq_SG_D_2_58af0 : Inport  Port=4
  State_psi_kq_SG_D_2_220dd : Inport  Port=5
  State_psi_q_SG_D_2_ffa91 : Inport  Port=6
  State_psi_gq_SG_D_2_c3a0a : Inport  Port=7
  State_psi_kq_SG_D_2_f5814 : Inport  Port=8
  State_psi_q_SG_D_2_8da15 : Inport  Port=9
  Add_097f1 : Sum
  Add_192a9 : Sum
  Add_263c1 : Sum
  Add_28e23 : Sum
  Add_5b11c : Sum
  Add_7138e : Sum
  Add_7e8a8 : Sum
  Add_d0e13 : Sum
  Add_d301e : Sum
  Add_e5b11 : Sum
  Add_e7dc4 : Sum
  Add_f2f46 : Sum
  Constant_-1_1fff4 : Constant  Value=-1
  Constant_-1_20f19 : Constant  Value=-1
  Constant_-1_3053f : Constant  Value=-1
  Constant_-1_6eb41 : Constant  Value=-1
  Constant_-1_8ed3a : Constant  Value=-1
  Constant_-1_ce113 : Constant  Value=-1
  Constant_-1_ce553 : Constant  Value=-1
  Constant_-1_cfd53 : Constant  Value=-1
  Constant_-1_d4d78 : Constant  Value=-1
  Constant_-1_fe51a : Constant  Value=-1
  Constant_2.0_23e3e : Constant  Value=2.0
  Constant_T_qd_b419f : Constant  Value=T_qd
  Constant_x_l_07f16 : Constant  Value=x_l
  Constant_x_l_17f69 : Constant  Value=x_l
  Constant_x_l_183ee : Constant  Value=x_l
  Constant_x_l_463e2 : Constant  Value=x_l
  Constant_x_l_7767e : Constant  Value=x_l
  Constant_x_l_7f296 : Constant  Value=x_l
  Constant_x_l_81d37 : Constant  Value=x_l
  Constant_x_l_94a18 : Constant  Value=x_l
  Constant_x_q_57059 : Constant  Value=x_q
  Constant_x_qd_2c20b : Constant  Value=x_qd
  Constant_x_qd_3e174 : Constant  Value=x_qd
  Constant_x_qd_43b99 : Constant  Value=x_qd
  Constant_x_qd_6a7a8 : Constant  Value=x_qd
  Constant_x_qd_6de9a : Constant  Value=x_qd
  Constant_x_qd_70e22 : Constant  Value=x_qd
  Constant_x_qd_8de2c : Constant  Value=x_qd
  Constant_x_qd_9a010 : Constant  Value=x_qd
  Constant_x_qd_a93cd : Constant  Value=x_qd
  Constant_x_qd_d7869 : Constant  Value=x_qd
  Constant_x_qdd_19ad3 : Constant  Value=x_qdd
  Constant_x_qdd_4abf0 : Constant  Value=x_qdd
  Constant_x_qdd_9c8cf : Constant  Value=x_qdd
  Constant_x_qdd_a0ac9 : Constant  Value=x_qdd
  Constant_x_qdd_b1d81 : Constant  Value=x_qdd
  Constant_x_qdd_d2fef : Constant  Value=x_qdd
  Constant_x_qdd_fcefd : Constant  Value=x_qdd
  Divide_06716 : Product  Inputs=*/
  Divide_1102a : Product  Inputs=*/
  Divide_721c2 : Product  Inputs=*/
  Divide_73421 : Product  Inputs=*/
  Divide_7963b : Product  Inputs=*/
  Divide_a59fc : Product  Inputs=*/
  Divide_c73ba : Product  Inputs=*/
  Divide_ca635 : Product  Inputs=*/
  Power_1085d : Math  Operator=pow
  Product_0484c : Product
  Product_21c16 : Product
  Product_3e470 : Product
  Product_59afe : Product
  Product_5a520 : Product
  Product_5b94e : Product
  Product_5dcf2 : Product
  Product_602b6 : Product
  Product_62fcf : Product
  Product_99e80 : Product
  Product_b0a2f : Product
  Product_b317f : Product
  Product_bbb55 : Product
  Product_ccfaa : Product
  Product_d2bae : Product
  Product_e85c7 : Product
  Product_f4e6a : Product
  Subtract_03ccb : Sum  Inputs=+-
  Subtract_2b99b : Sum  Inputs=+-
  Subtract_36f9e : Sum  Inputs=+-
  Subtract_67942 : Sum  Inputs=+-
  Subtract_7b83e : Sum  Inputs=+-
  Subtract_99c95 : Sum  Inputs=+-
  Subtract_aa6fa : Sum  Inputs=+-
  Subtract_bc9b3 : Sum  Inputs=+-
  Blockout_d_psi_gq_SG_D_2_29e5c : Outport
  wires:
  Constant_x_l_07f16/1 -> Product_0484c/2
  Constant_x_l_81d37/1 -> Product_62fcf/2
  Constant_x_qd_43b99/1 -> Subtract_99c95/1
  Constant_x_l_463e2/1 -> Product_bbb55/2
  Constant_x_qdd_b1d81/1 -> Subtract_03ccb/2
  Constant_-1_8ed3a/1 -> Product_3e470/1
  Constant_-1_20f19/1 -> Product_21c16/1
  State_psi_gq_SG_D_2_c98fa/1 -> Add_e5b11/1
  Constant_x_qdd_fcefd/1 -> Subtract_99c95/2
  Constant_x_qd_6de9a/1 -> Subtract_03ccb/1
  Constant_x_l_17f69/1 -> Product_3e470/2
  Constant_x_l_94a18/1 -> Product_21c16/2
  Product_3e470/1 -> Add_d301e/1
  Product_21c16/1 -> Add_28e23/1
  Constant_x_l_7f296/1 -> Product_59afe/2
  Constant_x_l_183ee/1 -> Product_d2bae/2
  Constant_x_qd_a93cd/1 -> Add_d301e/2
  Constant_x_qdd_d2fef/1 -> Add_28e23/2
  Constant_-1_3053f/1 -> Product_59afe/1
  Constant_x_qd_6a7a8/1 -> Add_d0e13/2
  Constant_x_qdd_9c8cf/1 -> Add_263c1/2
  State_psi_gq_SG_D_2_58af0/1 -> Product_99e80/1
  Add_d301e/1 -> Divide_721c2/2
  Add_28e23/1 -> Product_99e80/2
  Constant_x_qd_d7869/1 -> Subtract_36f9e/2
  Product_59afe/1 -> Add_192a9/1
  Constant_x_qd_70e22/1 -> Add_192a9/2
  State_psi_kq_SG_D_2_220dd/1 -> Product_b0a2f/1
  Divide_1102a/1 -> Subtract_aa6fa/1
  Subtract_99c95/1 -> Product_b0a2f/2
  Product_99e80/1 -> Divide_1102a/1
  Add_192a9/1 -> Divide_1102a/2
  Add_7e8a8/1 -> Product_5a520/2
  Product_b0a2f/1 -> Divide_721c2/1
  Constant_-1_ce553/1 -> Product_d2bae/1
  Divide_721c2/1 -> Subtract_aa6fa/2
  Constant_-1_1fff4/1 -> Product_0484c/1
  Constant_-1_cfd53/1 -> Product_62fcf/1
  Product_d2bae/1 -> Add_097f1/1
  Constant_x_qdd_a0ac9/1 -> Subtract_2b99b/2
  Constant_x_qd_2c20b/1 -> Add_097f1/2
  Subtract_aa6fa/1 -> Add_7e8a8/1
  Constant_-1_6eb41/1 -> Product_bbb55/1
  State_psi_q_SG_D_2_ffa91/1 -> Add_7e8a8/2
  Product_0484c/1 -> Add_d0e13/1
  Product_62fcf/1 -> Add_263c1/1
  Constant_-1_fe51a/1 -> Product_e85c7/1
  Product_5a520/1 -> Divide_c73ba/1
  Constant_x_l_7767e/1 -> Product_e85c7/2
  Product_f4e6a/1 -> Add_7138e/2
  Constant_x_qd_3e174/1 -> Subtract_2b99b/1
  Add_097f1/1 -> Product_5a520/1
  State_psi_gq_SG_D_2_c3a0a/1 -> Product_b317f/1
  Add_d0e13/1 -> Divide_73421/2
  Add_263c1/1 -> Product_b317f/2
  Product_e85c7/1 -> Add_e7dc4/1
  Constant_x_qd_9a010/1 -> Add_e7dc4/2
  State_psi_kq_SG_D_2_f5814/1 -> Product_5b94e/1
  Subtract_2b99b/1 -> Product_5b94e/2
  Divide_73421/1 -> Subtract_7b83e/2
  State_psi_kq_SG_D_2_803f1/1 -> Add_e5b11/2
  Product_5b94e/1 -> Divide_73421/1
  Constant_x_qdd_4abf0/1 -> Divide_c73ba/2
  Product_b317f/1 -> Divide_a59fc/1
  Add_e7dc4/1 -> Divide_a59fc/2
  Constant_-1_d4d78/1 -> Product_602b6/1
  Subtract_03ccb/1 -> Product_602b6/2
  Add_e5b11/1 -> Subtract_bc9b3/1
  Divide_c73ba/1 -> Subtract_bc9b3/2
  Product_bbb55/1 -> Add_f2f46/1
  Constant_x_qd_8de2c/1 -> Add_f2f46/2
  Divide_a59fc/1 -> Subtract_7b83e/1
  Product_602b6/1 -> Product_5dcf2/1
  Subtract_bc9b3/1 -> Product_5dcf2/2
  Add_f2f46/1 -> Power_1085d/1
  Constant_2.0_23e3e/1 -> Power_1085d/2
  Subtract_7b83e/1 -> Add_5b11c/1
  State_psi_q_SG_D_2_8da15/1 -> Add_5b11c/2
  Product_5dcf2/1 -> Divide_7963b/1
  Power_1085d/1 -> Divide_7963b/2
  Add_5b11c/1 -> Divide_ca635/1
  Constant_x_qdd_19ad3/1 -> Divide_ca635/2
  Constant_x_q_57059/1 -> Subtract_36f9e/1
  Divide_7963b/1 -> Subtract_67942/1
  Divide_ca635/1 -> Subtract_67942/2
  Divide_06716/1 -> Blockout_d_psi_gq_SG_D_2_29e5c/1
  Constant_-1_ce113/1 -> Product_ccfaa/1
  State_psi_gq_SG_D_2_87c46/1 -> Product_ccfaa/2
  Subtract_36f9e/1 -> Product_f4e6a/1
  Subtract_67942/1 -> Product_f4e6a/2
  Product_ccfaa/1 -> Add_7138e/1
  Add_7138e/1 -> Divide_06716/1
  Constant_T_qd_b419f/1 -> Divide_06716/2

== system case5/SG_D_2/d_psi_kq_SG_D_2_block ==
  note: d_psi_kq_SG_D_2 in case5
      | $-\frac{\psi _{\mathrm{gq},\mathrm{SG},D,2}+\psi _{\mathrm{kq},\mathrm{SG},D,2}+\frac{\left(x_{l}-x_{\mathrm{qd}}\right)\,\left(\psi _{q,\mathrm{SG},D,2}+\frac{\psi _{\mathrm{gq},\mathrm{SG},D,2}\,\left(x_{l}-x_{\mathrm{qdd}}\right)}{x_{l}-x_{\mathrm{qd}}}+\frac{\psi _{\mathrm{kq},\mathrm{SG},D,2}\,\left(x_{\mathrm{qd}}-x_{\mathrm{qdd}}\right)}{x_{l}-x_{\mathrm{qd}}}\right)}{x_{\mathrm{qdd}}}}{T_{\mathrm{qdd}}}$
      | Automatically generated on 2025-10-31 19:11:19 .
  State_psi_gq_SG_D_2_a995b : Inport
  State_psi_kq_SG_D_2_e8f3b : Inport  Port=2
  State_psi_gq_SG_D_2_50e2d : Inport  Port=3
  State_psi_kq_SG_D_2_80926 : Inport  Port=4
  State_psi_q_SG_D_2_342e1 : Inport  Port=5
  Add_0be58 : Sum
  Add_29be4 : Sum
  Add_3ec7e : Sum
  Add_971b1 : Sum
  Add_b0b93 : Sum
  Add_d3a29 : Sum
  Constant_-1_12e3a : Constant  Value=-1
  Constant_-1_13ae4 : Constant  Value=-1
  Constant_-1_68c7a : Constant  Value=-1
  Constant_-1_74188 : Constant  Value=-1
  Constant_-1_e3183 : Constant  Value=-1
  Constant_T_qdd_dc328 : Constant  Value=T_qdd
  Constant_x_l_710f0 : Constant  Value=x_l
  Constant_x_l_ae6dd : Constant  Value=x_l
  Constant_x_l_cc06b : Constant  Value=x_l
  Constant_x_l_ec336 : Constant  Value=x_l
  Constant_x_qd_0db5c : Constant  Value=x_qd
  Constant_x_qd_5fe60 : Constant  Value=x_qd
  Constant_x_qd_ac464 : Constant  Value=x_qd
  Constant_x_qd_bdb7a : Constant  Value=x_qd
  Constant_x_qdd_0bc51 : Constant  Value=x_qdd
  Constant_x_qdd_952ea : Constant  Value=x_qdd
  Constant_x_qdd_d405d : Constant  Value=x_qdd
  Divide_44808 : Product  Inputs=*/
  Divide_8ed1e : Product  Inputs=*/
  Divide_dc47c : Product  Inputs=*/
  Divide_e126f : Product  Inputs=*/
  Product_49a98 : Product
  Product_62856 : Product
  Product_6ee13 : Product
  Product_98e94 : Product
  Product_a6831 : Product
  Product_aa80f : Product
  Product_f9799 : Product
  Product_ff053 : Product
  Subtract_8b43e : Sum  Inputs=+-
  Subtract_b582a : Sum  Inputs=+-
  Subtract_e6ffd : Sum  Inputs=+-
  Blockout_d_psi_kq_SG_D_2_70fc6 : Outport
  wires:
  State_psi_kq_SG_D_2_e8f3b/1 -> Subtract_8b43e/2
  Constant_-1_74188/1 -> Product_aa80f/1
  Constant_-1_e3183/1 -> Product_ff053/1
  Constant_x_l_710f0/1 -> Product_ff053/2
  Constant_x_qdd_0bc51/1 -> Add_971b1/2
  Constant_x_l_ec336/1 -> Product_aa80f/2
  Constant_x_qd_0db5c/1 -> Subtract_e6ffd/1
  Constant_T_qdd_dc328/1 -> Divide_44808/2
  Constant_-1_68c7a/1 -> Product_62856/1
  Product_ff053/1 -> Add_971b1/1
  Constant_x_qdd_d405d/1 -> Subtract_e6ffd/2
  Constant_x_l_ae6dd/1 -> Product_62856/2
  Divide_44808/1 -> Blockout_d_psi_kq_SG_D_2_70fc6/1
  State_psi_gq_SG_D_2_50e2d/1 -> Product_6ee13/1
  Add_971b1/1 -> Product_6ee13/2
  Product_aa80f/1 -> Add_0be58/1
  Constant_x_qd_5fe60/1 -> Add_0be58/2
  Product_49a98/1 -> Divide_dc47c/1
  State_psi_kq_SG_D_2_80926/1 -> Product_a6831/1
  Subtract_e6ffd/1 -> Product_a6831/2
  Product_62856/1 -> Add_d3a29/1
  Constant_x_qd_ac464/1 -> Add_d3a29/2
  Product_a6831/1 -> Divide_8ed1e/1
  Product_6ee13/1 -> Divide_e126f/1
  Add_0be58/1 -> Divide_e126f/2
  Add_d3a29/1 -> Divide_8ed1e/2
  State_psi_q_SG_D_2_342e1/1 -> Add_b0b93/2
  Constant_-1_12e3a/1 -> Product_f9799/1
  Constant_x_l_cc06b/1 -> Product_f9799/2
  Divide_e126f/1 -> Subtract_b582a/1
  Divide_8ed1e/1 -> Subtract_b582a/2
  Product_f9799/1 -> Add_29be4/1
  Constant_x_qd_bdb7a/1 -> Add_29be4/2
  Subtract_b582a/1 -> Add_b0b93/1
  Constant_x_qdd_952ea/1 -> Divide_dc47c/2
  Constant_-1_13ae4/1 -> Product_98e94/1
  State_psi_gq_SG_D_2_a995b/1 -> Product_98e94/2
  Add_29be4/1 -> Product_49a98/1
  Add_b0b93/1 -> Product_49a98/2
  Product_98e94/1 -> Subtract_8b43e/1
  Subtract_8b43e/1 -> Add_3ec7e/1
  Divide_dc47c/1 -> Add_3ec7e/2
  Add_3ec7e/1 -> Divide_44808/1

== system case5/SG_D_2/d_psi_q_SG_D_2_block ==
  note: d_psi_q_SG_D_2 in case5
      | $2\,\pi \,f_{0}\,\left(v_{d,\mathrm{SG},D,2}\,\cos\left(\theta _{\mathrm{SG},D,2}\right)+v_{q,\mathrm{SG},D,2}\,\sin\left(\theta _{\mathrm{SG},D,2}\right)-\frac{R_{a}\,\left(\psi _{q,\mathrm{SG},D,2}+\frac{\psi _{\mathrm{gq},\mathrm{SG},D,2}\,\left(x_{l}-x_{\mathrm{qdd}}\right)}{x_{l}-x_{\mathrm{qd}}}+\frac{\psi _{\mathrm{kq},\mathrm{SG},D,2}\,\left(x_{\mathrm{qd}}-x_{\mathrm{qdd}}\right)}{x_{l}-x_{\mathrm{qd}}}\right)}{x_{\mathrm{qdd}}}-\frac{\psi _{d,\mathrm{SG},D,2}\,w_{\mathrm{SG},D,2}}{2\,f_{0}\,\pi }\right)$
      | Automatically generated on 2025-10-31 19:10:59 .
  State_psi_gq_SG_D_2_56d9a : Inport
  State_psi_kq_SG_D_2_66775 : Inport  Port=2
  State_psi_q_SG_D_2_48ee2 : Inport  Port=3
  Input_v_d_SG_D_2_6ca72 : Inport  Port=4
  State_theta_SG_D_2_953f6 : Inport  Port=5
  Input_v_q_SG_D_2_c1f9e : Inport  Port=6
  State_theta_SG_D_2_428e6 : Inport  Port=7
  State_psi_d_SG_D_2_a68ec : Inport  Port=8
  State_w_SG_D_2_ff297 : Inport  Port=9
  Add_42fda : Sum
  Add_6b2b5 : Sum
  Add_a40fa : Sum
  Add_b8587 : Sum
  Add_cedcf : Sum
  Constant_-1_5608d : Constant  Value=-1
  Constant_-1_6c9b4 : Constant  Value=-1
  Constant_-1_f7872 : Constant  Value=-1
  Constant_-2.0_32133 : Constant  Value=-2.0
  Constant_2.0_82335 : Constant  Value=2.0
  Constant_R_a_92f82 : Constant  Value=R_a
  Constant_f0_95229 : Constant  Value=f0
  Constant_f0_b0605 : Constant  Value=f0
  Constant_pi_1eedc : Constant  Value=pi
  Constant_pi_d98c1 : Constant  Value=pi
  Constant_x_l_1e216 : Constant  Value=x_l
  Constant_x_l_4f518 : Constant  Value=x_l
  Constant_x_l_6433a : Constant  Value=x_l
  Constant_x_qd_7775d : Constant  Value=x_qd
  Constant_x_qd_8b846 : Constant  Value=x_qd
  Constant_x_qd_8ea1e : Constant  Value=x_qd
  Constant_x_qdd_3d8ce : Constant  Value=x_qdd
  Constant_x_qdd_820db : Constant  Value=x_qdd
  Constant_x_qdd_f68a2 : Constant  Value=x_qdd
  Divide_2d835 : Product  Inputs=*/
  Divide_376ae : Product  Inputs=*/
  Divide_70c42 : Product  Inputs=*/
  Divide_e634e : Product  Inputs=*/
  MathFunc_cos_7f299 : Trigonometry  Operator=cos
  MathFunc_sin_f13ba : Trigonometry
  Product_017c0 : Product
  Product_424d1 : Product
  Product_49f5c : Product
  Product_5a243 : Product
  Product_7efc9 : Product
  Product_951ef : Product
  Product_ab076 : Product
  Product_b89ea : Product
  Product_bcf43 : Product
  Product_cbe93 : Product
  Product_d5df8 : Product
  Product_d81ca : Product
  Product_ebdd7 : Product
  Product_ff936 : Product
  Subtract_3ad7c : Sum  Inputs=+-
  Subtract_b2138 : Sum  Inputs=+-
  Subtract_ec7a0 : Sum  Inputs=+-
  Subtract_f6370 : Sum  Inputs=+-
  Blockout_d_psi_q_SG_D_2_3921f : Outport
  wires:
  Constant_x_qdd_3d8ce/1 -> Subtract_3ad7c/2
  Constant_x_l_4f518/1 -> Product_424d1/2
  Constant_-1_6c9b4/1 -> Product_ff936/1
  Constant_x_l_1e216/1 -> Product_ff936/2
  Product_ff936/1 -> Add_b8587/1
  Constant_pi_d98c1/1 -> Product_017c0/2
  State_psi_gq_SG_D_2_56d9a/1 -> Product_ebdd7/1
  Constant_x_l_6433a/1 -> Product_cbe93/2
  State_w_SG_D_2_ff297/1 -> Product_d5df8/2
  Constant_x_qd_8b846/1 -> Add_42fda/2
  Constant_x_qdd_820db/1 -> Add_b8587/2
  Constant_2.0_82335/1 -> Product_017c0/1
  Constant_-1_f7872/1 -> Product_cbe93/1
  Constant_x_qd_7775d/1 -> Subtract_3ad7c/1
  Constant_-1_5608d/1 -> Product_424d1/1
  State_psi_q_SG_D_2_48ee2/1 -> Add_cedcf/2
  Add_b8587/1 -> Product_ebdd7/2
  Product_017c0/1 -> Product_ab076/1
  Product_cbe93/1 -> Add_a40fa/1
  Constant_pi_1eedc/1 -> Product_b89ea/2
  Constant_f0_b0605/1 -> Product_ab076/2
  Constant_x_qd_8ea1e/1 -> Add_a40fa/2
  State_psi_kq_SG_D_2_66775/1 -> Product_d81ca/1
  Subtract_3ad7c/1 -> Product_d81ca/2
  Product_424d1/1 -> Add_42fda/1
  Input_v_q_SG_D_2_c1f9e/1 -> Product_49f5c/1
  Product_ebdd7/1 -> Divide_e634e/1
  Product_ab076/1 -> Divide_2d835/2
  Add_a40fa/1 -> Divide_e634e/2
  Product_d81ca/1 -> Divide_376ae/1
  Add_42fda/1 -> Divide_376ae/2
  Divide_e634e/1 -> Subtract_b2138/1
  State_theta_SG_D_2_953f6/1 -> MathFunc_cos_7f299/1
  Divide_376ae/1 -> Subtract_b2138/2
  Subtract_b2138/1 -> Add_cedcf/1
  MathFunc_cos_7f299/1 -> Product_7efc9/2
  Constant_R_a_92f82/1 -> Product_5a243/1
  Add_cedcf/1 -> Product_5a243/2
  State_theta_SG_D_2_428e6/1 -> MathFunc_sin_f13ba/1
  Product_5a243/1 -> Divide_70c42/1
  Product_b89ea/1 -> Product_951ef/1
  Product_49f5c/1 -> Subtract_f6370/2
  Constant_x_qdd_f68a2/1 -> Divide_70c42/2
  Input_v_d_SG_D_2_6ca72/1 -> Product_7efc9/1
  Add_6b2b5/1 -> Product_bcf43/2
  Divide_70c42/1 -> Subtract_ec7a0/1
  Product_7efc9/1 -> Subtract_ec7a0/2
  MathFunc_sin_f13ba/1 -> Product_49f5c/2
  Product_bcf43/1 -> Blockout_d_psi_q_SG_D_2_3921f/1
  State_psi_d_SG_D_2_a68ec/1 -> Product_d5df8/1
  Constant_-2.0_32133/1 -> Product_b89ea/1
  Product_951ef/1 -> Product_bcf43/1
  Subtract_ec7a0/1 -> Subtract_f6370/1
  Product_d5df8/1 -> Divide_2d835/1
  Constant_f0_95229/1 -> Product_951ef/2
  Subtract_f6370/1 -> Add_6b2b5/1
  Divide_2d835/1 -> Add_6b2b5/2

== system case5/SG_D_2/d_theta_SG_D_2_block ==
  note: d_theta_SG_D_2 in case5
      | $w_{\mathrm{SG},D,2}-2\,\pi \,f_{0}$
      | Automatically generated on 2025-10-31 19:11:26 .
  State_w_SG_D_2_4ff61 : Inport
  Add_b58ef : Sum
  Constant_-2.0_f0373 : Constant  Value=-2.0
  Constant_f0_17114 : Constant  Value=f0
  Constant_pi_7b554 : Constant  Value=pi
  Product_aea88 : Product
  Product_ffd51 : Product
  Blockout_d_theta_SG_D_2_f9fe2 : Outport
  wires:
  Constant_-2.0_f0373/1 -> Product_ffd51/1
  Constant_pi_7b554/1 -> Product_ffd51/2
  Add_b58ef/1 -> Blockout_d_theta_SG_D_2_f9fe2/1
  Product_ffd51/1 -> Product_aea88/1
  Constant_f0_17114/1 -> Product_aea88/2
  Product_aea88/1 -> Add_b58ef/1
  State_w_SG_D_2_4ff61/1 -> Add_b58ef/2
